simulink model "testemplanner_cs"  (R2020a)
settings: Solver=ode5  StartTime=0.0  StopTime=24  FixedStep=1/1000  RelTol=1e-3
PreLoadFcn:
  | mbxruntime.callbacks.PreLoadFcn(bdroot);
PostLoadFcn:
  | mbxruntime.callbacks.PostLoadFcn(bdroot);
InitFcn:
  | mbxruntime.callbacks.InitFcn(bdroot);
StartFcn:
  | mbxruntime.callbacks.StartFcn(bdroot);
StopFcn:
  | mbxruntime.callbacks.StopFcn(bdroot);
model workspace (MAT data in the model file):
  mbox_table : object (value not decoded)
  model_closed = 0
  sim_status = 0
values from neighbouring files (symbols this model uses):
  c_factor = 43.75    [emplanner_init.m]
  cf = -175016    [emplanner_init.m]
  cr = -130634    [emplanner_init.m]
  global_path_x = [0.057304 1.05668625507 2.05480936558 3.05165624935 4.04722112279 5.04150235808 6.03449985569 7.02621407764 8.01664569183 9.00579544113 9.99366409523 10.9802524329 ... (3001 elements, 3001x1)]    [global_path.mat]
  global_path_y = [8.29 8.29 8.29 8.29 8.29 8.29 8.29 8.29 8.29 8.29 8.29 8.29 ... (3001 elements, 3001x1)]    [global_path.mat]
  KD_PID_distance = 0.0    (= 0)    [emplanner_init.m]
  KD_PID_speed = 0    [emplanner_init.m]
  KI_PID_distance = 0.0    (= 0)    [emplanner_init.m]
  KI_PID_speed = 0    [emplanner_init.m]
  KP_PID_distance = 0.5    [emplanner_init.m]
  KP_PID_speed = 1.8    [emplanner_init.m]
  la = 1.265    [emplanner_init.m]
  lb = 2.947-1.265    (= 1.682)    [emplanner_init.m]
  LQR_K1 = k(:,1)'    [emplanner_init.m]
  LQR_K2 = k(:,2)'    [emplanner_init.m]
  LQR_K3 = k(:,3)'    [emplanner_init.m]
  LQR_K4 = k(:,4)'    [emplanner_init.m]
  m = 2020    [emplanner_init.m]
  rack_displacement = [-39.14 , -37.2 , -35.29 , -33.43 , -31.6 , -29.81 , -28.06 , -26.34 , -24.66 ,      -23.01 , -21.38 , -19.79 , -18.23 , -16.69 , -15.18 , -13.7 , -12.23 , -10.8 , -9.38 , -7.98 ,     -6.61 , -5.25 , -3.91 , -2.59 , -1.29 , 0 , 1.27 , 2.54 , 3.78 , 5.02 , 6.24 , 7.46 , 8.66 ,      9.86 , 11.05 , 12.24 , 13.41 , 14.59 , 15.76 , 16.92 , 18.09 , 19.25 , 20.42 , 21.59 , 22.76 ,      23.93 , 25.11 , 26 ...(+26 chars)    [emplanner_init.m]
  right_wheel_ground = [-70 ,-67.2 , -64.4 , -61.6 , -58.8 , -56 , -53.2 , -50.4 , -47.6 , -44.8 , -42 ,      -39.2 , -36.4 , -33.6 , -30.8 , -28 , -25.2 , -22.4 , -19.6 , -16.8 , -14 , -11.2 , -8.4 , -5.6 ,      -2.8 , 0 , 2.8 , 5.6 , 8.4 , 11.2 , 14 , 16.8 , 19.6 , 22.4 , 25.2 , 28 , 30.8 , 33.6 , 36.4 ,      39.2 , 42 , 44.8 , 47.6 , 50.4 , 53.2 , 56 , 58.8 , 61.6 , 64.4 , 67.2 , 70 ]    [emplanner_init.m]
  vx_break_point = zeros(1,5000)    [emplanner_init.m]
undefined symbols (not defined in the file or in its folder): aubr, DiscIntNeverNeededParam, tablebr, vubr
libraries: PreScanSimulinkLibrary x9, Solver_SF x1, simulink_extras x1
(part 6 of 9)

== matlab function testemplanner_cs/Audi_A8_Sedan_1/decision&planning module/EM_planner1/simple speed qp planning ==
  data: plan_start_s_dot input; s_init output; plan_start_s_dot2 input; s_end input; recommend_T input; s_dot_init output; s_dot2_init output; relative_time_init output
function [s_init,s_dot_init,s_dot2_init,relative_time_init] = fcn(plan_start_s_dot,plan_start_s_dot2,s_end,recommend_T)
%简单速度二次规划
coder.extrinsic("quadprog")
n = 51;
s_init = zeros(n,1);
s_dot_init = zeros(n,1);
s_dot2_init = zeros(n,1);
relative_time_init = zeros(n,1);

Aeq = zeros(3*n,2*n - 2);
beq = zeros(2*n - 2,1);
lb = ones(3*n,1);
ub = lb;
dt = recommend_T/(n-1);
A_sub =[1,0;
        dt,1;
        (1/3)*dt^2,(1/2)*dt;
        -1,0;
        0,-1;
        (1/6)*dt^2,dt/2];
for i = 1:n - 1
    Aeq(3*i-2:3*i+3,2*i-1:2*i) = A_sub;
end

for i = 1:n
   lb(3*i - 2) = -inf;
   lb(3*i - 1) = 0;
   lb(3*i) = -8;
   ub(3*i - 2) = inf;
   ub(3*i - 1) = 50;
   ub(3*i) = 2;
end
lb(1) = 0;
lb(2) = plan_start_s_dot;
lb(3) = plan_start_s_dot2;
ub(1) = lb(1);
ub(2) = lb(2);
ub(3) = lb(3);
lb(3*n - 2) = s_end;
ub(3*n - 2) = s_end;
A3 = zeros(3*n,3*n);
A4 = zeros(3*n,n - 1);
A4_sub =[0;0;1;0;0;-1];
for i = 1:n - 1
   A3(3*i,3*i) = 1;
   A4(3*i-2:3*i+3,i:i) = A4_sub;
end
A3(3*n,3*n) = 1;
H = A3 + 100*(A4*A4');
H = 2*H;
f = zeros(3*n,1);
X = quadprog(H,f,[],[],Aeq',beq,lb,ub);
for i = 1:n
   s_init(i) = X(3*i - 2);
   s_dot_init(i) = X(3*i - 1);
   s_dot2_init(i) = X(3*i);
   relative_time_init(i) = (i - 1)*dt;
end

== matlab function testemplanner_cs/Audi_A8_Sedan_1/decision&planning module/EM_planner1/stitch trajectory ==
  data: trajectory_x input; trajectory_x_final output; trajectory_y input; trajectory_heading input; trajectory_kappa input; trajectory_speed input; trajectory_accel input; trajectory_time input; stitch_x input; stitch_y input; stitch_heading input; stitch_kappa input; stitch_speed input; stitch_accel input; stitch_time input; trajectory_y_final output; trajectory_heading_final output; trajectory_kappa_final output; trajectory_speed_final output; trajectory_accel_final output; trajectory_time_final output
function [trajectory_x_final,trajectory_y_final,trajectory_heading_final,trajectory_kappa_final,trajectory_speed_final,trajectory_accel_final,trajectory_time_final] = fcn(trajectory_x,trajectory_y,trajectory_heading,trajectory_kappa,trajectory_speed,trajectory_accel,trajectory_time,...
    stitch_x,stitch_y,stitch_heading,stitch_kappa,stitch_speed,stitch_accel,stitch_time)

n=401+20;

trajectory_x_final=zeros(n,1);
trajectory_y_final=zeros(n,1);
trajectory_heading_final=zeros(n,1);
trajectory_kappa_final=zeros(n,1);
trajectory_speed_final=zeros(n,1);
trajectory_accel_final=zeros(n,1);
trajectory_time_final=zeros(n,1);



trajectory_x_final=[stitch_x;trajectory_x];
trajectory_y_final=[stitch_y;trajectory_y];
trajectory_heading_final=[stitch_heading;trajectory_heading];
trajectory_kappa_final=[stitch_kappa;trajectory_kappa];
trajectory_speed_final=[stitch_speed;trajectory_speed];
trajectory_accel_final=[stitch_accel;trajectory_accel];
trajectory_time_final=[stitch_time;trajectory_time];
end

== matlab function testemplanner_cs/Audi_A8_Sedan_1/decision&planning module/referenceline provider/calc path heading and kappa ==
  data: path_x input; path_heading output; path_y input; path_kappa output
function [path_heading,path_kappa] = fcn(path_x,path_y)
%%函数，已知路径的坐标点，计算路径的航向角和曲率
dx=diff(path_x);
dy=diff(path_y);
path_heading_init1=atan2(dy,dx);
for i=1:length(path_heading_init1)
    if path_heading_init1(i)<0
        path_heading_init1(i)=path_heading_init1(i)+2*pi;
    end
end
path_heading=[path_heading_init1;path_heading_init1(end)];
d_heading=sin(diff(path_heading));

ds=sqrt(dx.^2+dy.^2);

path_kappa1=d_heading./ds;
path_kappa=[path_kappa1;path_kappa1(end)];

== matlab function testemplanner_cs/Audi_A8_Sedan_1/decision&planning module/EM Planner/Index to s ==
  data: path_x input; index2s output; path_y input; origin_point_x input; origin_point_y input; origin_match_point_index input
function index2s = fcn(path_x,path_y,origin_point_x,origin_point_y,origin_match_point_index)
    
%作用：求出frenet坐标系下的点在世界坐标系下通过index所对应的s值，即index2s
%输入：参考线、frenet坐标原点的坐标，frenet坐标原点所对应的匹配点的index
%输出：index2s：index和s之间的对应关系

%首先定义index2s数组
n=181;
index2s=zeros(181,1);

%首先计算以path起点为原点的index2s值
for i=2:n
    index2s(i)=sqrt((path_x(i)-path_x(i-1))^2+(path_y(i)-path_y(i-1))^2)+index2s(i-1);
end

%再计算从path起点到匹配点的距离S0，用上面计算的index2s减去S0即可得出真实的index2s
%s_temp =  index2s(origin_match_point_index);
%调用函数，计算路径起点的index所对应的弧长s
s = CalcSfromIndex(path_x,path_y,origin_point_x,origin_point_y,origin_match_point_index,index2s);  
%用当前点到坐标原点的s减去路径起点到坐标原点的S，就是最终的距离路径起点的s
index2s=index2s-s*ones(n,1);
end
 function s=CalcSfromIndex(ref_path_x,ref_path_y,match_point_x,match_point_y,match_point_index,index2s)   %使用一个函数来计算index所对应的S值
%%首先判断原点是在匹配点前还是匹配点后，通过向量的内积来进行判断
s_temp =  index2s(match_point_index);
vector1=[match_point_x-ref_path_x(match_point_index);match_point_y-ref_path_y(match_point_index)];
%考虑匹配点在路径终点的情况，不在终点就是匹配点和下一个点作为方向向量，如果是终点则使用匹配点和上一个点作为方向向量
if match_point_index<length(ref_path_x)
    vector2=[ref_path_x(match_point_index+1)-ref_path_x(match_point_index);ref_path_y(match_point_index+1)-ref_path_y(match_point_index)];
else
     vector2=[ref_path_x(match_point_index)-ref_path_x(match_point_index-1);ref_path_y(match_point_index)-ref_path_y(match_point_index-1)];
end
result=vector1'*vector2;    
if result >0 %原点在匹配点后，加上这个距离
    s=s_temp+sqrt(vector1'*vector1);
else        %原点在匹配点前，减去这个距离
    s=s_temp-sqrt(vector1'*vector1);
end
end

== matlab function testemplanner_cs/Audi_A8_Sedan_1/decision&planning module/EM Planner/MATLAB Function5 ==
  data: x_set input; match_point_index_set output; y_set input; frenet_path_x input; frenet_path_y input; frenet_path_heading input; frenet_path_kappa input; proj_x_set output; proj_y_set output; proj_heading_set output; proj_kappa_set output
function [match_point_index_set,proj_x_set, proj_y_set,proj_heading_set,proj_kappa_set] = ...
    fcn(x_set,y_set,frenet_path_x,frenet_path_y,frenet_path_heading,frenet_path_kappa)
%该函数将批量计算x_set，y_set中的xy，在frenet_path下的投影的信息
%输入 x_set,y_set，待投影的点的集合
%x_set,y_set,frenet_path_x,frenet_path_y,frenet_path_heading,frenet_path_kappa
%曲线在直角坐标系下的x，y，heading，kappa
%输出：match_point_index_set 匹配点在frenet_path下的编号的集合(即从全局路径第一个点开始数，第几个点是匹配点)
%     proj_x y heading kappa 投影的x,y,heading,kappa的集合

% 由于事先不知道x_set中到底有多少个点需要投影，因此事先声明一个最大的数量的点作为缓冲
n = 128;
% 并且由于不知道投影点的个数，所以也不知道输出的个数，因此输出也要做缓冲，用nan表示不存在的点
% 输出最多输出128个
% 输出初始化
match_point_index_set = ones(n,1) * nan;
proj_x_set = ones(n,1) * nan;
proj_y_set = ones(n,1) * nan;
proj_heading_set = ones(n,1) * nan;
proj_kappa_set = ones(n,1) * nan;

%找匹配点，需要利用上一个周期的结果作为下一个周期遍历的起点，因此需要声明两个全局变量
persistent is_first_run;
persistent pre_match_point_index_set;
persistent pre_frenet_path_x;
persistent pre_frenet_path_y;
persistent pre_frenet_path_heading;
persistent pre_frenet_path_kappa;
%算法主函数入口

if isempty(is_first_run)
    %该if分支表示函数首次运行
    is_first_run = 0;
    pre_frenet_path_x = frenet_path_x;
    pre_frenet_path_y = frenet_path_y;
    pre_frenet_path_heading = frenet_path_heading;
    pre_frenet_path_kappa = frenet_path_kappa;
    %要记录首次运行计算的匹配点的结果供下个周期运行，先初始化
    pre_match_point_index_set = ones(n,1) * nan;
    %对x_set,y_set的点做遍历，找到他们的匹配点
    for i = 1 : length(x_set)
        if isnan(x_set(i))
            break;
        end
        %首次运行时，没有任何提示，只能从frenet path的第一个点开始找
        start_search_index = 1;
        % 声明increase_count，用于表示在遍历时distance连续增加的个数
        increase_count = 0;
        % 开始遍历
        min_distance = inf;
        for j = start_search_index : length(frenet_path_x)
            distance = (x_set(i) - frenet_path_x(j))^2 + (y_set(i) - frenet_path_y(j))^2;
            if distance < min_distance
                min_distance = distance;
                match_point_index_set(i) = j;
                increase_count = 0;
            else
                increase_count = increase_count + 1;
            end
            %如果distance连续增加50次就不要再遍历了，节省时间
            if increase_count > 50
                break;
            end
        end
        
        %如何通过匹配点计算投影点，请参见《自动驾驶控制算法第七讲》
        %或《自动驾驶决策规划算法》第一章第三节
        
        %取出匹配点的编号
        match_point_index = match_point_index_set(i);
        %取出匹配点的信息
        match_point_x = frenet_path_x(match_point_index);
        match_point_y = frenet_path_y(match_point_index);
        match_point_heading = frenet_path_heading(match_point_index);
        match_point_kappa = frenet_path_kappa(match_point_index);
        %计算匹配点的方向向量与法向量
        vector_match_point = [match_point_x;match_point_y];
        vector_match_point_direction = [cos(match_point_heading);sin(match_point_heading)];
        %声明待投影点的位矢
        vector_r = [x_set(i);y_set(i)];
        
       %通过匹配点计算投影点
       vector_d = vector_r - vector_match_point;
       ds = vector_d' * vector_match_point_direction;
       vector_proj_point = vector_match_point + ds * vector_match_point_direction;
       proj_heading = match_point_heading + match_point_kappa * ds;
       proj_kappa = match_point_kappa;
       %计算结果输出
       proj_x_set(i) = vector_proj_point(1);
       proj_y_set(i) = vector_proj_point(2);
       proj_heading_set(i) = proj_heading;
       proj_kappa_set(i) = proj_kappa;
    end
    %匹配点的计算结果保存，供下一个周期使用
    pre_match_point_index_set = match_point_index_set;
else
    %此if分支表示不是首次运行
    
    %对每个x_set上的点做处理
    for i = 1 : length(x_set)
        %不是首次运行，对于点x_set(i),y_set(i)来说,start_search_index =
        %pre_match_point_index_set(i)
        start_search_index = pre_match_point_index_set(i);%上个周期匹配点的编号作为本周期搜索的起点
        % 声明increase_count，用于表示在遍历时distance连续增加的个数
        %%%%%%%%%
        %对于障碍物检测而言，当感知第一次检测到障碍物时，算法并不是首次运行，此时 
        %pre_match_point_index_set的值是nan，如果还用上一时刻的结果作为本周期搜索的起点
        %必然会出问题，所以要修改
        % 声明increase_count_limit
        increase_count_limit = 5;
        if isnan(start_search_index)
            %没有上个周期的结果，那就不能只检查5次了
            increase_count_limit = 50;
            %搜索起点也要设为1
            start_search_index = 1;
        end
        increase_count = 0;
        % 开始遍历
        %这里多一个步骤，判断遍历的方向
        %计算上个周期匹配点的位矢
        vector_pre_match_point = [pre_frenet_path_x(start_search_index);pre_frenet_path_y(start_search_index)];
        vector_pre_match_point_direction = ...
            [cos(pre_frenet_path_heading(start_search_index));sin(pre_frenet_path_heading(start_search_index))];
        %判断遍历的方向
        flag = ([x_set(i);y_set(i)] - vector_pre_match_point)' * vector_pre_match_point_direction;
        min_distance = inf;
        if flag > 0.001
            for j = start_search_index : length(frenet_path_x)
                distance = (x_set(i) - frenet_path_x(j))^2 + (y_set(i) - frenet_path_y(j))^2;
                if distance < min_distance
                    min_distance = distance;
                    match_point_index_set(i) = j;
                    increase_count = 0;
                else
                    increase_count = increase_count + 1;
                end
                %如果distance连续增加increase_count_limit次就不要再遍历了，节省时间
                if increase_count > increase_count_limit
                    break;
                end
            end
        elseif flag < - 0.001
            for j = start_search_index : -1 : 1
                distance = (x_set(i) - frenet_path_x(j))^2 + (y_set(i) - frenet_path_y(j))^2;
                if distance < min_distance
                    min_distance = distance;
                    match_point_index_set(i) = j;
                    increase_count = 0;
                else
                    increase_count = increase_count + 1;
                end
                %如果distance连续增加increase_count_limit次就不要再遍历了，节省时间
                if increase_count > increase_count_limit
                    break;
                end
            end
        else
            match_point_index_set(i) = start_search_index;
        end
        
        %如何通过匹配点计算投影点，请参见《自动驾驶控制算法第七讲》
        %或《自动驾驶决策规划算法》第一章第三节
        
        %取出匹配点的编号
        match_point_index = match_point_index_set(i);
        %取出匹配点的信息
        match_point_x = frenet_path_x(match_point_index);
        match_point_y = frenet_path_y(match_point_index);
        match_point_heading = frenet_path_heading(match_point_index);
        match_point_kappa = frenet_path_kappa(match_point_index);
        %计算匹配点的方向向量与法向量
        vector_match_point = [match_point_x;match_point_y];
        vector_match_point_direction = [cos(match_point_heading);sin(match_point_heading)];
        %声明待投影点的位矢
        vector_r = [x_set(i);y_set(i)];
        
       %通过匹配点计算投影点
       vector_d = vector_r - vector_match_point;
       ds = vector_d' * vector_match_point_direction;
       vector_proj_point = vector_match_point + ds * vector_match_point_direction;
       proj_heading = match_point_heading + match_point_kappa * ds;
       proj_kappa = match_point_kappa;
       %计算结果输出
       proj_x_set(i) = vector_proj_point(1);
       proj_y_set(i) = vector_proj_point(2);
       proj_heading_set(i) = proj_heading;
       proj_kappa_set(i) = proj_kappa;
  
    end
    %匹配点的计算结果保存，供下一个周期使用
    pre_match_point_index_set = match_point_index_set;
    pre_frenet_path_x = frenet_path_x;
    pre_frenet_path_y = frenet_path_y;
    pre_frenet_path_heading = frenet_path_heading;
    pre_frenet_path_kappa = frenet_path_kappa;
end

== matlab function testemplanner_cs/Audi_A8_Sedan_1/decision&planning module/referenceline provider/generate referenceline from global path ==
  data: host_match_point_index input; referenceline_x_init output; path_x input; path_y input; referenceline_y_init output
function [referenceline_x_init,referenceline_y_init] = fcn(host_match_point_index,path_x,path_y)
%根据匹配点提取参考线
%往前取30个点，往后取150个点。
%如果不够的话进行补齐


host_match_point_index_init=host_match_point_index(1);%取匹配点的第一个元素作为匹配点的序号，适用于获得车辆投影点的情况
start_index=-1;%初始化参考线起始点位置序号
end_index=-1;%初始化参考线终点位置序号
%一般来讲从匹配点向前寻找30个点，向后寻找150个点。
if host_match_point_index_init< 31    %如果向前寻找的点不够30个，则选取最初的180个点
    start_index=1;
elseif host_match_point_index_init> length(path_x)-150 %如果向后寻找的点不够150个，则选取最后的180个点
    
    start_index=length(path_x)-180;
else                                                 %其他情况下则是向前选取30个点，向后选取150个点
    start_index=host_match_point_index_init-30;
    
end
referenceline_x_init=path_x(start_index:start_index+180);             %提取参考线x坐标
referenceline_y_init=path_y(start_index:start_index+180);             %提取参考线y坐标

== matlab function testemplanner_cs/Audi_A8_Sedan_1/decision&planning module/EM Planner/Frenet2Cart ==
  data: s_set input; x_set output; l_set input; dl_set input; ddl_set input; frenet_s input; frenet_l input; frenet_heading input; frenet_kappa input; index2s input; y_set output; heading_set output; kappa_set output
function [x_set,y_set,heading_set,kappa_set] = fcn(s_set,l_set,dl_set,ddl_set,frenet_s,frenet_l,frenet_heading,frenet_kappa,index2s)

%%作用：实现frenet坐标转换为笛卡尔坐标，进行控制.整个流程是先根据s求匹配点的x,y，再根据ds求投影点的x，y,再根据dl求要转换点的x,y
%%输入：frenet坐标下路径的s，l,dl,ddl;参考线的s,l,heading,kappa以及index2s

%%输出：路径在笛卡尔坐标系下的x,y,heading,kappa

%不知道要转换多少个点，因此进行缓冲

n=128;
%初始化输出
x_set=ones(n,1)*nan;
y_set=ones(n,1)*nan;
heading_set=ones(n,1)*nan;
kappa_set=ones(n,1)*nan;
for i=1:length(s_set)
    if isnan(s_set(i))
        break;
    end
    %写一个函数，用来计算路径s,l所对应的投影点的直角坐标系x，y，heading，kappa
    [proj_x,proj_y,proj_heading,proj_kappa]=calcProjPoint(s_set(i),frenet_s,frenet_l,frenet_heading,frenet_kappa,index2s);
    nor=[-sin(proj_heading);cos(proj_heading)];
    point_cert=[proj_x;proj_y]+l_set(i)*nor;
    x_set(i)=point_cert(1);
    y_set(i)=point_cert(2);
    heading_set(i) = proj_heading + atan(dl_set(i)/(1 - proj_kappa * l_set(i)));
    % 近似认为 kappa' == 0,frenet转cartesian公式，见第一章第三节评论区的链接
    kappa_set(i) = ((ddl_set(i) + proj_kappa * dl_set(i) * tan(heading_set(i) - proj_heading)) * ...
        (cos(heading_set(i) - proj_heading)^2)/(1 - proj_kappa * l_set(i)) + proj_kappa) * ...
        cos(heading_set(i) - proj_heading)/(1 - proj_kappa * l_set(i));
    
end
end


function  [proj_x,proj_y,proj_heading,proj_kappa]=calcProjPoint(s,frenet_x,frenet_y,frenet_heading,frenet_kappa,index2s)
   
    match_point_index = 1;
    while index2s(match_point_index) < s
        match_point_index = match_point_index + 1;
    end
    ds=s-index2s(match_point_index);
    tor=[cos(frenet_heading(match_point_index));sin(frenet_heading(match_point_index))];
    point=[frenet_x((match_point_index));frenet_y((match_point_index))]+ds*tor;
    proj_x=point(1);
    proj_y=point(2);
    proj_heading=frenet_heading((match_point_index))+ds*frenet_kappa(match_point_index);
    proj_kappa=frenet_kappa(match_point_index);
    end

== matlab function testemplanner_cs/Audi_A8_Sedan_1/decision&planning module/referenceline provider/reference_line_smooth ==
  data: referenceline_x_init input; referenceline_x output; referenceline_y_init input; pre_referenceline_x input; pre_referenceline_y input; w_ref_cost input; w_smooth_cost input; w_length_cost input; referenceline_x_lb input; referenceline_x_ub input; referenceline_y_lb input; referenceline_y_ub input; referenceline_y output
function [referenceline_x,referenceline_y] = fcn(referenceline_x_init,referenceline_y_init,pre_referenceline_x,pre_referenceline_y,w_ref_cost,w_smooth_cost,w_length_cost,referenceline_x_lb,referenceline_x_ub,referenceline_y_lb,referenceline_y_ub)
coder.extrinsic('quadprog');
%%此函数功能是利用二次规划的方法进行参考线的平滑

%输入：原始参考线点集
%输出：平滑后的参考线点集
%cost function =
%w1*((xi-xiref)^2+(yi-yiref)^2)+w2*((x（i-1）+x（i+1）-2xi)^2+(y（i-1）+y（i+1）-2yi)^2)+w3*((x（i+1）-xi)^2+(y（i+1）-yi)^2)

%首先确定数据维数
n=181;
persistent is_first_run
persistent pre_reference_x
persistent pre_reference_y
 
% if isempty(is_first_run)
%     is_first_run=0;
% %根据二次规划 1/2x'Hx+f'x=min
% %                Ax<=b
%  %               lb=<x,+yb
%  
%  %首先定义矩阵A1,A2,A3
%  A1=zeros(2*n-4,2*n);%平滑代价系数矩阵
%  A2=zeros(2*n-2,2*n);%紧凑代价系数矩阵
%  A3=eye(2*n,2*n);%几何相似代价系数矩阵
%  
%  M=zeros(2*n,1);
%  lb=M;
%  ub=M;
%  for i=1:n
%      M(2*i-1)=reference_line_x_init(i);
%      M(2*i)=reference_line_y_init(i);
%      lb(2*i-1)=reference_line_x_init(i)+reference_line_x_lb;
%      lb(2*i)=reference_line_y_init(i)+reference_line_y_lb;
%      ub(2*i-1)=reference_line_x_ub+reference_line_x_init(i);
%      ub(2*i)=reference_line_y_ub+reference_line_y_init(i);
%  end
% 
%  for j=1:2:2*n-5
%      A1(j,j)=1;
%      A1(j,j+2)=-2;
%      A1(j,j+4)=1;
%      A1(j+1,j+1)=1;
%      A1(j+1,j+3)=-2;
%      A1(j+1,j+5)=1;
%  end
%   for k=1:2:2*n-3
%      A2(k,k)=1;
%      A2(k,k+2)=-1;
%      A2(k+1,k+1)=1;
%      A2(k+1,k+3)=-1;
%   end
% H=w_smooth_cost*(A1'*A1)+w_length_cost*(A2'*A2)+w_ref_cost*A3; 
% H = 2 * H;
% X0 = M;
% f = -2*w_ref_cost*M;
if isempty(is_first_run)
    is_first_run = 0;
    A1=zeros(2*n-4,2*n);
    A2=zeros(2*n-2,2*n);
    f=zeros(n*2,1);
    lb=f;
    ub=f;
    for i=1:n
    f(2*i-1)=referenceline_x_init(i);
    f(2*i)=referenceline_y_init(i);
    lb(2*i-1)=referenceline_x_init(i)+referenceline_x_lb;
    lb(2*i)=referenceline_y_init(i)+referenceline_y_lb;
    ub(2*i-1)=referenceline_x_init(i)+referenceline_x_ub;
    ub(2*i)=referenceline_y_init(i)+referenceline_y_ub;
    end

    for i=1:2:2*n-5
    A1(i,i)=1;
    A1(i,i+2)=-2;
    A1(i,i+4)=1;
    A1(i+1,i+1)=1;
    A1(i+1,i+3)=-2;
    A1(i+1,i+5)=1; 
    end
    for i=1:2:2*n-3
    A2(i,i)=1;
    A2(i,i+2)=-1;    
    A2(i+1,i+1)=1;
    A2(i+1,i+3)=-1;  
    end
    A3=eye(2*n,2*n);
    H=w_smooth_cost*(A1'*A1)+w_length_cost*(A2'*A2)+w_ref_cost*A3;
    H=2*H;
    X0=f;
    f=-2*w_ref_cost*f;
    X=quadprog(H,f,[],[],[],[],lb,ub,X0);
    
%     x=zeros(n,1);
%     y=zeros(n,1);
%     for i=1:n
%         x(i)=X(2*i-1);
%         y(i)=X(2*i);
%     end
%     if isempty(is_first_run)
%     is_first_run = 0;
%     A1=zeros(2*n-4,2*n);
%     A2=zeros(2*n-2,2*n);
%     f=zeros(n*2,1);
%     lb=f;
%     ub=f;
%     for i=1:n
%     f(2*i-1)=referenceline_x_init(i);
%     f(2*i)=referenceline_y_init(i);
%     lb(2*i-1)=referenceline_x_init(i)+referenceline_x_lb;
%     lb(2*i)=referenceline_y_init(i)+referenceline_y_lb;
%     ub(2*i-1)=referenceline_x_init(i)+referenceline_x_ub;
%     ub(2*i)=referenceline_y_init(i)+referenceline_y_ub;
%     end

%     for i=1:2:2*n-5
%     A1(i,i)=1;
%     A1(i,i+2)=-2;
%     A1(i,i+4)=1;
%     A1(i+1,i+1)=1;
%     A1(i+1,i+3)=-2;
%     A1(i+1,i+5)=1; 
%     end
%     for i=1:2:2*n-3
%     A2(i,i)=1;
%     A2(i,i+2)=-1;    
%     A2(i+1,i+1)=1;
%     A2(i+1,i+3)=-1;  
%     end
%     A3=eye(2*n,2*n);
%     H=w_smooth_cost*(A1'*A1)+w_length_cost*(A2'*A2)+w_ref_cost*A3;
%     H=2*H;
%     X0=f;
%     f=-2*w_ref_cost*f;

%     X=quadprog(H,f,[],[],[],[],lb,ub,X0);
    x=zeros(n,1);
    y=zeros(n,1);

    for i=1:n
    x(i)=X(2*i-1);
    y(i)=X(2*i);
    end
    referenceline_x=x;
    referenceline_y=y;
    pre_reference_x=x;
    pre_reference_y=y;
else
    index=-1;
    new_reference_line_x=referenceline_x_init(1);
    new_reference_line_y=referenceline_y_init(1);
    for i=1:length(pre_referenceline_x)
        if (pre_referenceline_x(i)==new_reference_line_x)&&(pre_referenceline_y(i)==new_reference_line_y)
            index=i;
            break;
        end
    end
        if index==-1||index>6
            %首先定义矩阵A1,A2,A3
            A1=zeros(2*n-4,2*n);%平滑代价系数矩阵
            A2=zeros(2*n-2,2*n);%紧凑代价系数矩阵
            A3=eye(2*n,2*n);%几何相似代价系数矩阵
            
            M=zeros(2*n,1);
            lb=M;
            ub=M;
            for i=1:n
                M(2*i-1)=referenceline_x_init(i);
                M(2*i)=referenceline_y_init(i);
                lb(2*i-1)=referenceline_x_init(i)-referenceline_x_lb;
                lb(2*i)=referenceline_y_init(i)-referenceline_y_lb;
                ub(2*i-1)=referenceline_x_ub+referenceline_x_init(i);
                ub(2*i)=referenceline_y_ub+referenceline_y_init(i);
            end
            
            for i=1:2:2*n-5
                A1(i,i)=1;
                A1(i,i+2)=-2;
                A1(i,i+4)=1;
                A1(i+1,i+1)=1;
                A1(i+1,i+3)=-2;
                A1(i+1,i+5)=1;
            end
            for i=1:2:2*n-3
                A2(i,i)=1;
                A2(i,i+2)=-1;
                A2(i+1,i+1)=1;
                A2(i+1,i+3)=-1;
            end
            H=2*(w_smooth_cost*(A1'*A1)+w_length_cost*(A2'*A2)+w_ref_cost*A3);
            f = w_ref_cost*(-2*M);
            X=quadprog(H,f,[],[],[],[],lb,ub,M);
            x=zeros(n,1);
            y=zeros(n,1);
            for i=1:n
                x(i)=X(2*i-1);
                y(i)=X(2*i);
            end
            referenceline_x=x;
            referenceline_y=y;
            pre_reference_x=x;
            pre_reference_y=y;
        elseif index==1
            referenceline_x=pre_reference_x;
            referenceline_y=pre_reference_y;   
        else
            %开始进行轨迹拼接，但是拼接点的个数无法确定，先定义成6个,但因为要带上原有轨迹的两个点，所以是6+2个
            point_num=6+2;
            A1=zeros(2*point_num-4,2*point_num);%平滑代价系数矩阵
            A2=zeros(2*point_num-2,2*point_num);%紧凑代价系数矩阵
            A3=eye(2*point_num,2*point_num);%几何相似代价系数矩阵
              
            M=zeros(2*point_num,1);
            lb=M;
            ub=M;
            
            %要拼接的点个数是序号-1
            joint_num=index-1;
            M(1)=pre_reference_x(length(referenceline_x_init) - 1);
            M(2)=pre_reference_y(length(referenceline_x_init) - 1);
            M(3)=pre_reference_x(length(referenceline_x_init));
            M(4)=pre_reference_y(length(referenceline_x_init));
            lb(1)=M(1);
            lb(2)=M(2);
            lb(3)=M(3);
            lb(4)=M(4);
            ub(1)=M(1);
            ub(2)=M(2);
            ub(3)=M(3);
            ub(4)=M(4);
            %因为前面有joint_num个点是一样的，所以只需要平滑最后剩下的几个点即可
            start_index=length(referenceline_x_init)-joint_num;
            for i=1:joint_num
            M(2*i+3)=referenceline_x_init(start_index+i);
            M(2*i+4)=referenceline_y_init(start_index+i);
            lb(2*i+3)=referenceline_x_init(start_index+i)-referenceline_x_lb;
            lb(2*i+4)=referenceline_y_init(start_index+i)-referenceline_y_lb;
            ub(2*i+3)=referenceline_x_init(start_index+i)+referenceline_x_ub;
            ub(2*i+4)=referenceline_y_init(start_index+i)+referenceline_y_ub;
            end
             for i=1:2:2*(joint_num+2)-5
                A1(i,i)=1;
                A1(i,i+2)=-2;
                A1(i,i+4)=1;
                A1(i+1,i+1)=1;
                A1(i+1,i+3)=-2;
                A1(i+1,i+5)=1;
            end
            for i=1:2:2*(joint_num+2)-3
                A2(i,i)=1;
                A2(i,i+2)=-1;
                A2(i+1,i+1)=1;
                A2(i+1,i+3)=-1;
            end
            H=2*(w_smooth_cost*(A1'*A1)+w_length_cost*(A2'*A2)+w_ref_cost*(A3'*A3));
            f = w_ref_cost*(-2*M);
            X=quadprog(H,f,[],[],[],[],lb,ub,M);
            x=zeros(joint_num,1);
            y=zeros(joint_num,1);
            for i=1:joint_num
                x(i)=X(2*i+3);
                y(i)=X(2*i+4);
            end
            referenceline_x=zeros(n,1);
            referenceline_y=zeros(n,1);
            %进行轨迹拼接
            for i=1:length(referenceline_x_init)
                if i<=length(referenceline_x_init)-joint_num
                    referenceline_x(i)=pre_reference_x(i+joint_num);
                    referenceline_y(i)=pre_reference_y(i+joint_num);
                else
                    referenceline_x(i)=x(i-length(referenceline_x_init)+joint_num);
                    referenceline_y(i)=y(i-length(referenceline_x_init)+joint_num);
                end
            end
            
            pre_reference_x=referenceline_x;
            pre_reference_y=referenceline_y;
         
        end
end

== matlab function testemplanner_cs/Audi_A8_Sedan_1/control module2/MATLAB Function1 ==
  data: trajectory_x input; xr output; trajectory_y input; trajectory_heading input; trajectory_kappa input; trajectory_speed input; trajectory_accel input; trajectory_time input; current_time input; yr output; thetar output; kappar output; vr output; ar output
function [xr,yr,thetar,kappar,vr,ar] = fcn(trajectory_x,trajectory_y,trajectory_heading,...
    trajectory_kappa,trajectory_speed,trajectory_accel,trajectory_time,current_time)
% 该函数根据规划的轨迹计算出期望跟踪的点
% 由于控制也是有延迟，所以控制发出的期望跟踪的点是current_time + 0.01;
control_time = current_time + 0.01;
% 规划发出的轨迹有一部分是拼接的，在刚启动的时候，stitch_time = -1,因此要先把它去掉
start_index = 1;
while (trajectory_time(start_index) == -1)
    start_index = start_index + 1;
end
% 使用interp1插值计算得到xr yr thetar,kappar,vr,ar
% 由于interp1在端点会得到nan，因此需要防一手
% 解释，为什么需要trajectory_time(start_index) ~= 0
% 因为在刚启动时规划先执行(100ms)，当规划完毕的时候控制已经执行了10次
% 那么在最开始的时候，规划还没给结果是控制已经执行了10次，在这10次中控制跟踪的轨迹是空轨迹
% simulink 空轨迹表示为 0，0，0，0，0，0......,这样trajectory_time
% 也全是0，trajectory_time不单调递增
% 而interp1(x,y,x0)要求x必须要单调递增，否则会报错，所以当规划首次运行时控制需要执行下面这个else分支的代码，否则会报错
if control_time > trajectory_time(start_index) && trajectory_time(start_index) ~= 0
    xr = interp1(trajectory_time(start_index:end),trajectory_x(start_index:end),control_time);
    yr = interp1(trajectory_time(start_index:end),trajectory_y(start_index:end),control_time);
    thetar = interp1(trajectory_time(start_index:end),trajectory_heading(start_index:end),control_time);
    kappar = interp1(trajectory_time(start_index:end),trajectory_kappa(start_index:end),control_time);
    vr = interp1(trajectory_time(start_index:end),trajectory_speed(start_index:end),control_time);
    ar = interp1(trajectory_time(start_index:end),trajectory_accel(start_index:end),control_time);
else
    xr = trajectory_x(start_index);
    yr = trajectory_y(start_index);
    thetar = trajectory_heading(start_index);
    kappar = trajectory_kappa(start_index);
    vr = trajectory_speed(start_index);
    ar = trajectory_accel(start_index);
end

== matlab function testemplanner_cs/Audi_A8_Sedan_1/decision&planning module/EM Planner/calc plan start and stitch trajectory ==
  data: host_x input; plan_start_x output; host_y input; host_heading_xy input; host_vx input; host_vy input; host_ax input; host_ay input; pre_trajectory_x input; pre_trajectory_y input; pre_trajectory_heading input; pre_trajectory_kappa input; pre_trajectory_velocity input; pre_trajectory_accelerate input; pre_trajectory_time input; current_time input; plan_start_y output; plan_start_heading output; plan_start_kappa output; plan_start_vx output; plan_start_vy output; plan_start_ax output; plan_start_ay output; plan_start_time output; stitch_x output; stitch_y output; stitch_heading output; stitch_kappa output; stitch_velocity output; stitch_accelerate output; stitch_time output
function [plan_start_x,plan_start_y,plan_start_heading,plan_start_kappa,plan_start_vx,plan_start_vy,plan_start_ax,plan_start_ay,plan_start_time,stitch_x,stitch_y,...
    stitch_heading,stitch_kappa,stitch_velocity,stitch_accelerate,stitch_time] = fcn(host_x,host_y,host_heading_xy,host_vx,host_vy,host_ax,host_ay,pre_trajectory_x,pre_trajectory_y,...
    pre_trajectory_heading,pre_trajectory_kappa,pre_trajectory_velocity,pre_trajectory_accelerate,pre_trajectory_time,current_time)

%%作用：求得当前周期的规划起点，有两种方式，①一种方式是车辆当前位置与上一周期规划路径点相差较大，此时需要通过车辆动力学外推得到，②另一种方式是相差不大，直径将原有路径延长得到
%%输入：上一个周期规划出的路径的坐标点，航向，速度，加速度。车辆当前的坐标点、航向，速度，加速度，当前时间。
%%输出；规划起点的坐标点，航向，速度，加速度；待拼接轨迹的坐标点，航向，速度，加速度以及时间。

% 初始化待拼接轨迹，此轨迹主要用来进行拼接，加速计算过程，待拼接轨迹为计算的规划起点在原有轨迹上的位置向前取20个点，因此初始化一个20个点的数组
stitch_x=zeros(20,1);
stitch_y=zeros(20,1);
stitch_heading=zeros(20,1);
stitch_kappa=zeros(20,1);
stitch_velocity=zeros(20,1);
stitch_accelerate=zeros(20,1);
%时间初始化为-1，代表没有要拼接的轨迹
stitch_time=ones(20,1)*(-1);

%根据是否为第一次运行进行区分，
persistent is_first_run

if isempty(is_first_run)
    %算法首次运行，本来需要外推，但因为是首次运行就以车辆当前的位置作为规划起点
    is_first_run=0;
    plan_start_x=host_x;
    plan_start_y=host_y;
    plan_start_heading=host_heading_xy;
    plan_start_kappa=0;
    plan_start_vx=0;
    plan_start_vy=0;
    plan_start_ax=0;
    plan_start_ay=0;
    %规划起点时间戳为当前时间+100ms
    plan_start_time=current_time+0.1;
else
    %算法不是首次运行，可以正常运行
    
    %比较车辆当前实际位置与车辆规划位置的差别
    
    x_current=host_x;
    y_current=host_y;
    heading_current=host_heading_xy;
    kappa_current=0;%默认起点曲率为0
    %要转换为世界坐标系
    vx_current=host_vx*cos(heading_current)-host_vy*sin(heading_current);
    vy_current=host_vx*sin(heading_current)+host_vy*cos(heading_current);
    ax_current=host_ax*cos(heading_current)-host_ay*sin(heading_current);
    ay_current=host_ax*sin(heading_current)+host_ay*cos(heading_current);
    %接着遍历数组，求解根据规划，车辆当前应道在的位置
    dt=0.1;
    for i=1:length(pre_trajectory_time)-1
        if(pre_trajectory_time(i)<=current_time)&&(pre_trajectory_time(i+1)>current_time)
           break; 
        end
    end
    x_desire=pre_trajectory_x(i);
    y_desire=pre_trajectory_y(i);
    heading_desire=pre_trajectory_heading(i);
%     vx_desire=pre_trajectory_velocity*cos(pre_trajectory_heading(i));
%     vy_desire=pre_trajectory_velocity*sin(pre_trajectory_heading(i));
%     ax_desire=pre_trajectory_accelerate*cos(pre_trajectory_heading(i));
%     ay_desire=pre_trajectory_accelerate*sin(pre_trajectory_heading(i));
    
   %得到两个位置的误差
   %通过向量法计算误差
   %切向向量
   tor = [cos(heading_desire);sin(heading_desire)];
   %法向向量
   nor = [-sin(heading_desire);cos(heading_desire)];
   %两点向量
   error = [host_x;host_y]-[x_desire;y_desire];
   %纵向误差
   long_error = abs(error'*tor);
   %横向误差
   lat_error = abs(error'*nor);
   
   if (long_error>2.5)||(lat_error>0.5)   %控制误差过大，使用车辆动力学外推
        
        plan_start_x=x_current+vx_current*dt+0.5*ax_current*dt*dt;
        plan_start_y=y_current+vy_current*dt+0.5*ay_current*dt*dt;
        plan_start_kappa=kappa_current;
        plan_start_vx=vx_current+ax_current*dt;
        plan_start_vy=vy_current+ay_current*dt;
        plan_start_ax=ax_current;
        plan_start_ay=ay_current;
        plan_start_heading=atan2(plan_start_vy,plan_start_vx);
    %规划起点时间戳为当前时间+100ms
        plan_start_time=current_time+0.1;
        return;
   else     %控制误差不大，则利用上一个周期规划路径找点
       for j=i:length(pre_trajectory_time)-1
            if (pre_trajectory_time(j)<=current_time+0.1)&&(pre_trajectory_time(j+1)>current_time+0.1)
                break;
            end
       end
        plan_start_x=pre_trajectory_x(j);
        plan_start_y=pre_trajectory_y(j);
        plan_start_heading=pre_trajectory_heading(j);
        plan_start_kappa=pre_trajectory_kappa(j);
        plan_start_vx=pre_trajectory_velocity(j)*cos(plan_start_heading);
        plan_start_vy=pre_trajectory_velocity(j)*sin(plan_start_heading);
        % 注意，由于是做圆周运动，所以加速度要先按照切向和法相进行分解
         %切向向量
         tor = [cos(plan_start_heading);sin(plan_start_heading)];
         %法向向量
         nor = [-sin(plan_start_heading);cos(plan_start_heading)];
        tor_a=pre_trajectory_accelerate(j)*tor;        %切向加速度
        nor_a=pre_trajectory_velocity(j)^2*plan_start_kappa*nor; %法向加速度=v^2/r
        %分别将切向加速度和法向加速度的x，y分量相加就是ax和ay
        plan_start_ax=tor_a(1)+nor_a(1);
        plan_start_ay=tor_a(2)+nor_a(2);
    %规划起点时间戳为当前时间+100ms
        plan_start_time=pre_trajectory_time(j); 
         %下面开始进行轨迹拼接
         %当前节点是j，如果j大于20，则往前拼接20个点，如果j<20，则能拼几个点就拼几个点。从stitch最后一个点开始拼，没有拼上的点time为-1
         if j>=21
            stitch_x = pre_trajectory_x(j - 20:j-1);
            stitch_y = pre_trajectory_y(j - 20:j-1);
            stitch_heading = pre_trajectory_heading(j - 20:j-1);
            stitch_kappa = pre_trajectory_kappa(j - 20:j-1);
            stitch_velocity = pre_trajectory_velocity(j - 20:j-1);
            stitch_accelerate = pre_trajectory_accelerate(j - 20:j-1);
            stitch_time = pre_trajectory_time(j - 20:j-1);
         else
             for k=1:j-1
                 stitch_time(20+1-k)=pre_trajectory_time(j-k);
                 stitch_x(20+1-k)=pre_trajectory_x(j-k);
                 stitch_y(20+1-k)=pre_trajectory_y(j-k);
                 stitch_heading(20+1-k)=pre_trajectory_heading(j-k);
                 stitch_kappa(20+1-k)=pre_trajectory_kappa(j-k);
                 stitch_velocity(20+1-k) = pre_trajectory_velocity(j-k);
                 stitch_accelerate(20+1-k) = pre_trajectory_accelerate(j-k);
             end
         end
   end
%         j = j - 1;
%         if j >= 20
%             stitch_x = pre_trajectory_x(j - 19:j);
%             stitch_y = pre_trajectory_y(j - 19:j);
%             stitch_heading = pre_trajectory_heading(j - 19:j);
%             stitch_kappa = pre_trajectory_kappa(j - 19:j);
%             stitch_velocity = pre_trajectory_velocity(j - 19:j);
%             stitch_accelerate = pre_trajectory_accelerate(j - 19:j);
%             stitch_time = pre_trajectory_time(j - 19:j);
%         else
%             stitch_x(20 - j + 1:20) = pre_trajectory_x(1:j);
%             stitch_y(20 - j + 1:20) = pre_trajectory_y(1:j);
%             stitch_heading(20 - j + 1:20) = pre_trajectory_heading(1:j);
%             stitch_kappa(20 - j + 1:20) = pre_trajectory_kappa(1:j);
%             stitch_accelerate(20 - j + 1:20) = pre_trajectory_velocity(1:j);
%             stitch_accelerate(20 - j + 1:20) = pre_trajectory_accelerate(1:j);
%             stitch_time(20 - j + 1:20) = pre_trajectory_time(1:j);           
%         end   
%    end
%    
   
   
end

== matlab function testemplanner_cs/Audi_A8_Sedan_1/decision&planning module/EM Planner/stitch trajectory ==
  data: trajectory_x input; trajectory_x_final output; trajectory_y input; trajectory_heading input; trajectory_kappa input; trajectory_speed input; trajectory_accel input; trajectory_time input; stitch_x input; stitch_y input; stitch_heading input; stitch_kappa input; stitch_speed input; stitch_accel input; stitch_time input; trajectory_y_final output; trajectory_heading_final output; trajectory_kappa_final output; trajectory_speed_final output; trajectory_accel_final output; trajectory_time_final output
function [trajectory_x_final,trajectory_y_final,trajectory_heading_final,trajectory_kappa_final,trajectory_speed_final,trajectory_accel_final,trajectory_time_final] = fcn(trajectory_x,trajectory_y,trajectory_heading,trajectory_kappa,trajectory_speed,trajectory_accel,trajectory_time,...
    stitch_x,stitch_y,stitch_heading,stitch_kappa,stitch_speed,stitch_accel,stitch_time)

n=401+20;

trajectory_x_final=zeros(n,1);
trajectory_y_final=zeros(n,1);
trajectory_heading_final=zeros(n,1);
trajectory_kappa_final=zeros(n,1);
trajectory_speed_final=zeros(n,1);
trajectory_accel_final=zeros(n,1);
trajectory_time_final=zeros(n,1);



trajectory_x_final=[stitch_x;trajectory_x];
trajectory_y_final=[stitch_y;trajectory_y];
trajectory_heading_final=[stitch_heading;trajectory_heading];
trajectory_kappa_final=[stitch_kappa;trajectory_kappa];
trajectory_speed_final=[stitch_speed;trajectory_speed];
trajectory_accel_final=[stitch_accel;trajectory_accel];
trajectory_time_final=[stitch_time;trajectory_time];
end

== matlab function testemplanner_cs/Audi_A8_Sedan_1/decision&planning module/EM Planner/obs1/Cart2Frenet/CalcSL ==
  data: x_set input; y_set input; referenceline_x input; referenceline_y input; index2s input; plan_start_match_point_index input; plan_start_proj_x input; plan_start_proj_y input; plan_start_proj_heading input; plan_start_proj_kappa input; frenet_s_set output; frenet_l_set output
function [frenet_s_set,frenet_l_set] =fcn(x_set,y_set,referenceline_x,referenceline_y,index2s,plan_start_match_point_index,plan_start_proj_x,plan_start_proj_y,plan_start_proj_heading,plan_start_proj_kappa)
%作用：这是一个通用函数，计算输入的笛卡尔坐标点x,y在自然坐标（frenet）坐标系中的s和l
%输入:要计算的点集的x,y坐标，航向，曲率。他的投影点的x,y坐标，index2s数据，以及参考线数据
%输出：自然坐标系下的s和l
%首先对s和l做一个缓冲
frenet_s_set=ones(128,1)*nan;
frenet_l_set=ones(128,1)*nan;
%开始计算
for i=1:length(x_set)
if isnan(x_set(i))  %遇到空的跳出
    break;
end
%调用相关函数进行s的计算
frenet_s_set(i)=CalcSfromIndex(referenceline_x,referenceline_y,plan_start_proj_x(i),plan_start_proj_y(i),plan_start_match_point_index(i),index2s);

%进行l的计算
%先求自然坐标系的切向量和法向量
%切向量,没用到
%tor=[cos(plan_start_proj_heading(i));sin(plan_start_proj_heading(i))];
%法向量
nor=[-sin(plan_start_proj_heading(i));cos(plan_start_proj_heading(i))];
frenet_l_set(i)=[x_set(i)-plan_start_proj_x(i);y_set(i)-plan_start_proj_y(i)]'*nor;
end

end
function s=CalcSfromIndex(ref_path_x,ref_path_y,match_point_x,match_point_y,match_point_index,index2s)   %使用一个函数来计算index所对应的S值
%%首先判断原点是在匹配点前还是匹配点后，通过向量的内积来进行判断
s_temp =  index2s(match_point_index);
vector1=[match_point_x-ref_path_x(match_point_index);match_point_y-ref_path_y(match_point_index)];
%考虑匹配点在路径终点的情况，不在终点就是匹配点和下一个点作为方向向量，如果是终点则使用匹配点和上一个点作为方向向量
if match_point_index<length(ref_path_x)
    vector2=[ref_path_x(match_point_index+1)-ref_path_x(match_point_index);ref_path_y(match_point_index+1)-ref_path_y(match_point_index)];
else
     vector2=[ref_path_x(match_point_index)-ref_path_x(match_point_index-1);ref_path_y(match_point_index)-ref_path_y(match_point_index-1)];
end
result=vector1'*vector2;    
if result >0 %原点在匹配点后，加上这个距离
    s=s_temp+sqrt(vector1'*vector1);
else        %原点在匹配点前，减去这个距离
    s=s_temp-sqrt(vector1'*vector1);
end
end

== matlab function testemplanner_cs/Audi_A8_Sedan_1/decision&planning module/EM Planner/obs1/Cart2Frenet/CalcSL2 ==
  data: frenet_l_set input; ax_set input; ay_set input; s_dot_set input; dl_set input; plan_start_proj_heading input; plan_start_proj_kappa input; s_dot2_set output; l_dot2_set output; ddl_set output
function [ s_dot2_set, l_dot2_set,ddl_set]=fcn(frenet_l_set,ax_set,ay_set,s_dot_set,dl_set,plan_start_proj_heading,plan_start_proj_kappa)
%作用：通过之前计算得到的l，s_dot、dl值以及已知的ax，ay值，计算s_dot2,l_dot2,以及ddl
 %首先做一个缓冲
 n=128;
 s_dot2_set=ones(n,1)*nan;
 l_dot2_set=ones(n,1)*nan;
 ddl_set=ones(n,1)*nan;

 for i=1:length(frenet_l_set)
     if isnan(frenet_l_set(i))
         break;
     end
    %先求自然坐标系的切向量和法向量
%切向量
tor=[cos(plan_start_proj_heading(i));sin(plan_start_proj_heading(i))];
%法向量
nor=[-sin(plan_start_proj_heading(i));cos(plan_start_proj_heading(i))];

ah=[ax_set(i);ay_set(i)];
l_dot2_set(i)=ah'*nor- plan_start_proj_kappa(i) * (1 - plan_start_proj_kappa(i) * frenet_l_set(i)) * s_dot_set(i)^2;
s_dot2_set(i)=(1/(1 - plan_start_proj_kappa(i) * frenet_l_set(i)))* (ah' * tor + 2 * plan_start_proj_kappa(i) * dl_set(i) * s_dot_set(i)^2);

if abs(s_dot2_set(i))<1e-6
    ddl_set(i)=0;
else
    ddl_set(i)=(l_dot2_set(i) - dl_set(i)*s_dot2_set(i))/(s_dot_set(i)^2);
 end
end

== matlab function testemplanner_cs/Audi_A8_Sedan_1/decision&planning module/EM Planner/obs1/Cart2Frenet/Calcs_l_dot_dl ==
  data: frenet_l_set input; vx_set input; vy_set input; plan_start_proj_heading input; plan_start_proj_kappa input; s_dot_set output; l_dot_set output; dl_set output
function [ s_dot_set, l_dot_set,dl_set]=fcn(frenet_l_set,vx_set,vy_set,plan_start_proj_heading,plan_start_proj_kappa)
%作用：通过之前计算得到的s和l值以及计算的速度值，计算s_dot,l_dot,以及dl
 %首先做一个缓冲
 n=128;
 s_dot_set=ones(n,1)*nan;
 l_dot_set=ones(n,1)*nan;
 dl_set=ones(n,1)*nan;

 for i=1:length(frenet_l_set)
     if isnan(frenet_l_set(i))
         break;
     end
    %先求自然坐标系的切向量和法向量
%切向量
tor=[cos(plan_start_proj_heading(i));sin(plan_start_proj_heading(i))];
%法向量
nor=[-sin(plan_start_proj_heading(i));cos(plan_start_proj_heading(i))];

vh=[vx_set(i);vy_set(i)];
l_dot_set(i)=vh'*nor;
s_dot_set(i)=vh'*tor/(1-plan_start_proj_kappa(i)*frenet_l_set(i));

if abs(s_dot_set(i))<1e-6
    dl_set(i)=0;
else
    dl_set(i)=l_dot_set(i)/s_dot_set(i);
 end
end
